simulink model "FSAC2021_V1_Running"  (R2014a)
settings: Solver=FixedStepDiscrete  StartTime=0.0  StopTime=inf  FixedStep=0.0005  RelTol=1e-3
model workspace (MAT data in the model file):
  MCOS : class17 (value not decoded)
  MCOS : class17 (value not decoded)
  MCOS : class17 (value not decoded)
  MCOS : class17 (value not decoded)
  MCOS : class17 (value not decoded)
  MCOS : class17 (value not decoded)
  MCOS : class17 (value not decoded)
  MCOS : class17 (value not decoded)
  MCOS : class17 (value not decoded)
  MCOS : class17 (value not decoded)
  MCOS : class17 (value not decoded)
  MCOS : class17 (value not decoded)
  MCOS : class17 (value not decoded)
  MCOS : class17 (value not decoded)
  MCOS : class17 (value not decoded)
  MCOS : class17 (value not decoded)
  MCOS : class17 (value not decoded)
  MCOS : class17 (value not decoded)
  MCOS : class17 (value not decoded)
  BUZZER_START = 1
  MCOS : class17 (value not decoded)
  MCOS : class17 (value not decoded)
  MCOS : class17 (value not decoded)
  MCOS : class17 (value not decoded)
  MCOS : class17 (value not decoded)
  MCOS : class17 (value not decoded)
  MCOS : class17 (value not decoded)
  MCOS : class17 (value not decoded)
  MCOS : class17 (value not decoded)
  MCOS : class17 (value not decoded)
  MCOS : class17 (value not decoded)
  MCOS : class17 (value not decoded)
  MCOS : class17 (value not decoded)
  MCOS : class17 (value not decoded)
  MCOS : class17 (value not decoded)
  MCOS : class17 (value not decoded)
  MCOS : class17 (value not decoded)
  MCOS : class17 (value not decoded)
  MCOS : class17 (value not decoded)
  MCOS : class17 (value not decoded)
  MCOS : class17 (value not decoded)
  MCOS : class17 (value not decoded)
  MCOS : class17 (value not decoded)
  MCOS : class17 (value not decoded)
  MCOS : class17 (value not decoded)
  MCOS : class17 (value not decoded)
  MCOS : class17 (value not decoded)
  MCOS : class17 (value not decoded)
  MCOS : class17 (value not decoded)
  MCOS : class17 (value not decoded)
  MCOS : class17 (value not decoded)
  MCOS : class17 (value not decoded)
  MCOS : class17 (value not decoded)
  MCOS : class17 (value not decoded)
  MCOS : class17 (value not decoded)
  MCOS : class17 (value not decoded)
  MCOS : class17 (value not decoded)
  MCOS : class17 (value not decoded)
  Brake = 11
  MCOS : class17 (value not decoded)
  MCOS : class17 (value not decoded)
  MCOS : class17 (value not decoded)
  MCOS : class17 (value not decoded)
  MCOS : class17 (value not decoded)
  MCOS : class17 (value not decoded)
  MCOS : class17 (value not decoded)
  MCOS : class17 (value not decoded)
  Sensor_Acc_b = 101.85
  Sensor_Acc_k = -0.0185
  Str_Sen_Orig_Angle = -341
  MCOS : class17 (value not decoded)
  Tire_D = 0.47
  T = 0.05
libraries: simulink x402, ec55xxlib x134
(part 15 of 17)

== system FSAC2021_V1_Running/ROUTING/TO_DCAN/Subsystem/DIAG_SCU/Operation_Enabled ==
  Operation_Enabled : Inport
  Operation_EnabledRon : Rounding  Operator=round
  Operation_Enabled_1sat : Saturate  UpperLimit=16  LowerLimit=0
  Operation_Enabled_Convert : DataTypeConversion  OutDataTypeStr=uint8
  Operation_Enabled_Convert1 : DataTypeConversion  OutDataTypeStr=uint32
  Operation_Enabled_D : Product  Inputs=*/
  Operation_Enabled_F : Constant  OutDataTypeStr=single
  Operation_Enabled_L : simulink/Logic and Bit Operations/Bitwise Operator  logicop=AND  UseBitMask=on  BitMask=16  BitMaskRealWorld=Stored Integer
  Operation_Enabled_O : Constant  Value=0  OutDataTypeStr=single
  Operation_Enabled_S : ArithShift  BitShiftNumber=-4
  Operation_Enabled_sat : Saturate  UpperLimit=0  LowerLimit=0
  Operation_Enabled_st : Sum  Inputs=+-
  output5 : Outport
  wires:
  Operation_Enabled/1 -> Operation_Enabled_sat/1
  Operation_Enabled_sat/1 -> Operation_Enabled_st/1
  Operation_Enabled_O/1 -> Operation_Enabled_st/2
  Operation_Enabled_st/1 -> Operation_Enabled_D/1
  Operation_Enabled_F/1 -> Operation_Enabled_D/2
  Operation_Enabled_D/1 -> Operation_EnabledRon/1
  Operation_EnabledRon/1 -> Operation_Enabled_S/1
  Operation_Enabled_S/1 -> Operation_Enabled_1sat/1
  Operation_Enabled_1sat/1 -> Operation_Enabled_Convert1/1
  Operation_Enabled_Convert1/1 -> Operation_Enabled_L/1
  Operation_Enabled_L/1 -> Operation_Enabled_Convert/1
  Operation_Enabled_Convert/1 -> output5/1

== system FSAC2021_V1_Running/ROUTING/TO_DCAN/Subsystem/DIAG_SCU/Str_Ang ==
  Str_Ang : Inport
  Str_AngBitCov : DataTypeConversion  OutDataTypeStr=uint8
  Str_AngCOV : DataTypeConversion  OutDataTypeStr=uint8
  Str_AngRon : Rounding  Operator=round
  Str_Ang_1sat : Saturate  UpperLimit=65535  LowerLimit=0
  Str_Ang_And : simulink/Logic and Bit Operations/Bitwise Operator  logicop=AND  UseBitMask=off  NumInputPorts=2  BitMask=bin2dec('11011001')  BitMaskRealWorld=Stored Integer
  Str_Ang_And_C : Constant  Value=255  OutDataTypeStr=uint32
  Str_Ang_Convert : DataTypeConversion  OutDataTypeStr=uint32
  Str_Ang_D : Product  Inputs=*/
  Str_Ang_D1 : Product  Inputs=*/
  Str_Ang_F : Constant  OutDataTypeStr=single
  Str_Ang_L : simulink/Logic and Bit Operations/Bitwise Operator  logicop=AND  UseBitMask=on  BitMask=65535  BitMaskRealWorld=Stored Integer
  Str_Ang_O : Constant  Value=0  OutDataTypeStr=single
  Str_Ang_S : ArithShift
  Str_Ang_sat : Saturate  UpperLimit=65535  LowerLimit=0
  Str_Ang_st : Sum  Inputs=+-
  Str_Angoutput2_C : Constant  Value=256
  output2 : Outport
  output3 : Outport  Port=2
  wires:
  Str_Ang/1 -> Str_Ang_sat/1
  Str_Ang_sat/1 -> Str_Ang_st/1
  Str_Ang_O/1 -> Str_Ang_st/2
  Str_Ang_st/1 -> Str_Ang_D/1
  Str_Ang_F/1 -> Str_Ang_D/2
  Str_Ang_D/1 -> Str_AngRon/1
  Str_AngRon/1 -> Str_Ang_S/1
  Str_Ang_S/1 -> Str_Ang_1sat/1
  Str_Ang_1sat/1 -> Str_Ang_Convert/1
  Str_Ang_Convert/1 -> Str_Ang_L/1
  Str_Ang_L/1 -> Str_Ang_D1/1, Str_Ang_And/1
  Str_Angoutput2_C/1 -> Str_Ang_D1/2
  Str_Ang_D1/1 -> Str_AngCOV/1
  Str_AngCOV/1 -> output2/1
  Str_Ang_And_C/1 -> Str_Ang_And/2
  Str_Ang_And/1 -> Str_AngBitCov/1
  Str_AngBitCov/1 -> output3/1

== system FSAC2021_V1_Running/ROUTING/TO_DCAN/Subsystem/DIAG_SCU/Str_Curr_Error_Fault ==
  Str_Curr_Error_Fault : Inport
  Str_Curr_Error_FaultRon : Rounding  Operator=round
  Str_Curr_Error_Fault_1sat : Saturate  UpperLimit=32  LowerLimit=0
  Str_Curr_Error_Fault_Convert : DataTypeConversion  OutDataTypeStr=uint8
  Str_Curr_Error_Fault_Convert1 : DataTypeConversion  OutDataTypeStr=uint32
  Str_Curr_Error_Fault_D : Product  Inputs=*/
  Str_Curr_Error_Fault_F : Constant  OutDataTypeStr=single
  Str_Curr_Error_Fault_L : simulink/Logic and Bit Operations/Bitwise Operator  logicop=AND  UseBitMask=on  BitMask=32  BitMaskRealWorld=Stored Integer
  Str_Curr_Error_Fault_O : Constant  Value=0  OutDataTypeStr=single
  Str_Curr_Error_Fault_S : ArithShift  BitShiftNumber=-5
  Str_Curr_Error_Fault_sat : Saturate  UpperLimit=0  LowerLimit=0
  Str_Curr_Error_Fault_st : Sum  Inputs=+-
  output7 : Outport
  wires:
  Str_Curr_Error_Fault/1 -> Str_Curr_Error_Fault_sat/1
  Str_Curr_Error_Fault_sat/1 -> Str_Curr_Error_Fault_st/1
  Str_Curr_Error_Fault_O/1 -> Str_Curr_Error_Fault_st/2
  Str_Curr_Error_Fault_st/1 -> Str_Curr_Error_Fault_D/1
  Str_Curr_Error_Fault_F/1 -> Str_Curr_Error_Fault_D/2
  Str_Curr_Error_Fault_D/1 -> Str_Curr_Error_FaultRon/1
  Str_Curr_Error_FaultRon/1 -> Str_Curr_Error_Fault_S/1
  Str_Curr_Error_Fault_S/1 -> Str_Curr_Error_Fault_1sat/1
  Str_Curr_Error_Fault_1sat/1 -> Str_Curr_Error_Fault_Convert1/1
  Str_Curr_Error_Fault_Convert1/1 -> Str_Curr_Error_Fault_L/1
  Str_Curr_Error_Fault_L/1 -> Str_Curr_Error_Fault_Convert/1
  Str_Curr_Error_Fault_Convert/1 -> output7/1

== system FSAC2021_V1_Running/ROUTING/TO_DCAN/Subsystem/DIAG_SCU/Str_Current ==
  Str_Current : Inport
  Str_CurrentABS : Abs
  Str_CurrentCS : ArithShift  BitShiftNumber=-8
  Str_CurrentConS : Constant  OutDataTypeStr=single
  Str_CurrentCosR : Constant  Value=0  OutDataTypeStr=uint8
  Str_CurrentROP : RelationalOperator  Operator=<  OutDataTypeStr=boolean
  Str_CurrentRon : Rounding  Operator=round
  Str_CurrentSW : Switch  Criteria=u2 ~= 0
  Str_Current_1sat : Saturate  UpperLimit=255  LowerLimit=0
  Str_Current_Convert : DataTypeConversion  OutDataTypeStr=uint8
  Str_Current_Convert1 : DataTypeConversion  OutDataTypeStr=uint32
  Str_Current_D : Product  Inputs=*/
  Str_Current_F : Constant  OutDataTypeStr=single
  Str_Current_L : simulink/Logic and Bit Operations/Bitwise Operator  logicop=AND  UseBitMask=on  BitMask=255  BitMaskRealWorld=Stored Integer
  Str_Current_O : Constant  Value=0  OutDataTypeStr=single
  Str_Current_S : ArithShift
  Str_Current_sat : Saturate  UpperLimit=127  LowerLimit=-128
  Str_Current_st : Sum  Inputs=+-
  Str_Currentsubcon : Sum  Inputs=+-
  output4 : Outport
  wires:
  Str_Current/1 -> Str_Current_sat/1
  Str_Current_sat/1 -> Str_Current_st/1
  Str_Current_O/1 -> Str_Current_st/2
  Str_Current_st/1 -> Str_Current_D/1
  Str_Current_F/1 -> Str_Current_D/2
  Str_Current_D/1 -> Str_CurrentRon/1
  Str_CurrentRon/1 -> Str_CurrentROP/1, Str_CurrentABS/1, Str_CurrentSW/3
  Str_CurrentCosR/1 -> Str_CurrentROP/2
  Str_CurrentConS/1 -> Str_CurrentCS/1
  Str_CurrentCS/1 -> Str_Currentsubcon/1
  Str_CurrentABS/1 -> Str_Currentsubcon/2
  Str_Currentsubcon/1 -> Str_CurrentSW/1
  Str_CurrentROP/1 -> Str_CurrentSW/2
  Str_CurrentSW/1 -> Str_Current_S/1
  Str_Current_S/1 -> Str_Current_1sat/1
  Str_Current_1sat/1 -> Str_Current_Convert1/1
  Str_Current_Convert1/1 -> Str_Current_L/1
  Str_Current_L/1 -> Str_Current_Convert/1
  Str_Current_Convert/1 -> output4/1

== system FSAC2021_V1_Running/ROUTING/TO_DCAN/Subsystem/DIAG_SCU/Str_Deg ==
  Str_Deg : Inport
  Str_DegABS : Abs
  Str_DegCS : ArithShift  BitShiftNumber=-8
  Str_DegConS : Constant  OutDataTypeStr=single
  Str_DegCosR : Constant  Value=0  OutDataTypeStr=uint8
  Str_DegROP : RelationalOperator  Operator=<  OutDataTypeStr=boolean
  Str_DegRon : Rounding  Operator=round
  Str_DegSW : Switch  Criteria=u2 ~= 0
  Str_Deg_1sat : Saturate  UpperLimit=255  LowerLimit=0
  Str_Deg_Convert : DataTypeConversion  OutDataTypeStr=uint8
  Str_Deg_Convert1 : DataTypeConversion  OutDataTypeStr=uint32
  Str_Deg_D : Product  Inputs=*/
  Str_Deg_F : Constant  OutDataTypeStr=single
  Str_Deg_L : simulink/Logic and Bit Operations/Bitwise Operator  logicop=AND  UseBitMask=on  BitMask=255  BitMaskRealWorld=Stored Integer
  Str_Deg_O : Constant  Value=0  OutDataTypeStr=single
  Str_Deg_S : ArithShift
  Str_Deg_sat : Saturate  UpperLimit=120  LowerLimit=-120
  Str_Deg_st : Sum  Inputs=+-
  Str_Degsubcon : Sum  Inputs=+-
  output1 : Outport
  wires:
  Str_Deg/1 -> Str_Deg_sat/1
  Str_Deg_sat/1 -> Str_Deg_st/1
  Str_Deg_O/1 -> Str_Deg_st/2
  Str_Deg_st/1 -> Str_Deg_D/1
  Str_Deg_F/1 -> Str_Deg_D/2
  Str_Deg_D/1 -> Str_DegRon/1
  Str_DegRon/1 -> Str_DegROP/1, Str_DegABS/1, Str_DegSW/3
  Str_DegCosR/1 -> Str_DegROP/2
  Str_DegConS/1 -> Str_DegCS/1
  Str_DegCS/1 -> Str_Degsubcon/1
  Str_DegABS/1 -> Str_Degsubcon/2
  Str_Degsubcon/1 -> Str_DegSW/1
  Str_DegROP/1 -> Str_DegSW/2
  Str_DegSW/1 -> Str_Deg_S/1
  Str_Deg_S/1 -> Str_Deg_1sat/1
  Str_Deg_1sat/1 -> Str_Deg_Convert1/1
  Str_Deg_Convert1/1 -> Str_Deg_L/1
  Str_Deg_L/1 -> Str_Deg_Convert/1
  Str_Deg_Convert/1 -> output1/1

== system FSAC2021_V1_Running/ROUTING/TO_DCAN/Subsystem/DIAG_SCU/Str_Encoder_Error ==
  Str_Encoder_Error : Inport
  Str_Encoder_ErrorRon : Rounding  Operator=round
  Str_Encoder_Error_1sat : Saturate  UpperLimit=16  LowerLimit=0
  Str_Encoder_Error_Convert : DataTypeConversion  OutDataTypeStr=uint8
  Str_Encoder_Error_Convert1 : DataTypeConversion  OutDataTypeStr=uint32
  Str_Encoder_Error_D : Product  Inputs=*/
  Str_Encoder_Error_F : Constant  OutDataTypeStr=single
  Str_Encoder_Error_L : simulink/Logic and Bit Operations/Bitwise Operator  logicop=AND  UseBitMask=on  BitMask=16  BitMaskRealWorld=Stored Integer
  Str_Encoder_Error_O : Constant  Value=0  OutDataTypeStr=single
  Str_Encoder_Error_S : ArithShift  BitShiftNumber=-4
  Str_Encoder_Error_sat : Saturate  UpperLimit=0  LowerLimit=0
  Str_Encoder_Error_st : Sum  Inputs=+-
  output6 : Outport
  wires:
  Str_Encoder_Error/1 -> Str_Encoder_Error_sat/1
  Str_Encoder_Error_sat/1 -> Str_Encoder_Error_st/1
  Str_Encoder_Error_O/1 -> Str_Encoder_Error_st/2
  Str_Encoder_Error_st/1 -> Str_Encoder_Error_D/1
  Str_Encoder_Error_F/1 -> Str_Encoder_Error_D/2
  Str_Encoder_Error_D/1 -> Str_Encoder_ErrorRon/1
  Str_Encoder_ErrorRon/1 -> Str_Encoder_Error_S/1
  Str_Encoder_Error_S/1 -> Str_Encoder_Error_1sat/1
  Str_Encoder_Error_1sat/1 -> Str_Encoder_Error_Convert1/1
  Str_Encoder_Error_Convert1/1 -> Str_Encoder_Error_L/1
  Str_Encoder_Error_L/1 -> Str_Encoder_Error_Convert/1
  Str_Encoder_Error_Convert/1 -> output6/1

== system FSAC2021_V1_Running/ROUTING/TO_DCAN/Subsystem/DIAG_SCU/Str_Flash_Error ==
  Str_Flash_Error : Inport
  Str_Flash_ErrorRon : Rounding  Operator=round
  Str_Flash_Error_1sat : Saturate  UpperLimit=8  LowerLimit=0
  Str_Flash_Error_Convert : DataTypeConversion  OutDataTypeStr=uint8
  Str_Flash_Error_Convert1 : DataTypeConversion  OutDataTypeStr=uint32
  Str_Flash_Error_D : Product  Inputs=*/
  Str_Flash_Error_F : Constant  OutDataTypeStr=single
  Str_Flash_Error_L : simulink/Logic and Bit Operations/Bitwise Operator  logicop=AND  UseBitMask=on  BitMask=8  BitMaskRealWorld=Stored Integer
  Str_Flash_Error_O : Constant  Value=0  OutDataTypeStr=single
  Str_Flash_Error_S : ArithShift  BitShiftNumber=-3
  Str_Flash_Error_sat : Saturate  UpperLimit=0  LowerLimit=0
  Str_Flash_Error_st : Sum  Inputs=+-
  output6 : Outport
  wires:
  Str_Flash_Error/1 -> Str_Flash_Error_sat/1
  Str_Flash_Error_sat/1 -> Str_Flash_Error_st/1
  Str_Flash_Error_O/1 -> Str_Flash_Error_st/2
  Str_Flash_Error_st/1 -> Str_Flash_Error_D/1
  Str_Flash_Error_F/1 -> Str_Flash_Error_D/2
  Str_Flash_Error_D/1 -> Str_Flash_ErrorRon/1
  Str_Flash_ErrorRon/1 -> Str_Flash_Error_S/1
  Str_Flash_Error_S/1 -> Str_Flash_Error_1sat/1
  Str_Flash_Error_1sat/1 -> Str_Flash_Error_Convert1/1
  Str_Flash_Error_Convert1/1 -> Str_Flash_Error_L/1
  Str_Flash_Error_L/1 -> Str_Flash_Error_Convert/1
  Str_Flash_Error_Convert/1 -> output6/1

== system FSAC2021_V1_Running/ROUTING/TO_DCAN/Subsystem/DIAG_SCU/Str_I2t_Alarm ==
  Str_I2t_Alarm : Inport
  Str_I2t_AlarmRon : Rounding  Operator=round
  Str_I2t_Alarm_1sat : Saturate  UpperLimit=1  LowerLimit=0
  Str_I2t_Alarm_Convert : DataTypeConversion  OutDataTypeStr=uint8
  Str_I2t_Alarm_Convert1 : DataTypeConversion  OutDataTypeStr=uint32
  Str_I2t_Alarm_D : Product  Inputs=*/
  Str_I2t_Alarm_F : Constant  OutDataTypeStr=single
  Str_I2t_Alarm_L : simulink/Logic and Bit Operations/Bitwise Operator  logicop=AND  UseBitMask=on  BitMask=1  BitMaskRealWorld=Stored Integer
  Str_I2t_Alarm_O : Constant  Value=0  OutDataTypeStr=single
  Str_I2t_Alarm_S : ArithShift
  Str_I2t_Alarm_sat : Saturate  UpperLimit=0  LowerLimit=0
  Str_I2t_Alarm_st : Sum  Inputs=+-
  output5 : Outport
  wires:
  Str_I2t_Alarm/1 -> Str_I2t_Alarm_sat/1
  Str_I2t_Alarm_sat/1 -> Str_I2t_Alarm_st/1
  Str_I2t_Alarm_O/1 -> Str_I2t_Alarm_st/2
  Str_I2t_Alarm_st/1 -> Str_I2t_Alarm_D/1
  Str_I2t_Alarm_F/1 -> Str_I2t_Alarm_D/2
  Str_I2t_Alarm_D/1 -> Str_I2t_AlarmRon/1
  Str_I2t_AlarmRon/1 -> Str_I2t_Alarm_S/1
  Str_I2t_Alarm_S/1 -> Str_I2t_Alarm_1sat/1
  Str_I2t_Alarm_1sat/1 -> Str_I2t_Alarm_Convert1/1
  Str_I2t_Alarm_Convert1/1 -> Str_I2t_Alarm_L/1
  Str_I2t_Alarm_L/1 -> Str_I2t_Alarm_Convert/1
  Str_I2t_Alarm_Convert/1 -> output5/1

== system FSAC2021_V1_Running/ROUTING/TO_DCAN/Subsystem/DIAG_SCU/Str_I2t_Warning ==
  Str_I2t_Warning : Inport
  Str_I2t_WarningRon : Rounding  Operator=round
  Str_I2t_Warning_1sat : Saturate  UpperLimit=2  LowerLimit=0
  Str_I2t_Warning_Convert : DataTypeConversion  OutDataTypeStr=uint8
  Str_I2t_Warning_Convert1 : DataTypeConversion  OutDataTypeStr=uint32
  Str_I2t_Warning_D : Product  Inputs=*/
  Str_I2t_Warning_F : Constant  OutDataTypeStr=single
  Str_I2t_Warning_L : simulink/Logic and Bit Operations/Bitwise Operator  logicop=AND  UseBitMask=on  BitMask=2  BitMaskRealWorld=Stored Integer
  Str_I2t_Warning_O : Constant  Value=0  OutDataTypeStr=single
  Str_I2t_Warning_S : ArithShift  BitShiftNumber=-1
  Str_I2t_Warning_sat : Saturate  UpperLimit=0  LowerLimit=0
  Str_I2t_Warning_st : Sum  Inputs=+-
  output5 : Outport
  wires:
  Str_I2t_Warning/1 -> Str_I2t_Warning_sat/1
  Str_I2t_Warning_sat/1 -> Str_I2t_Warning_st/1
  Str_I2t_Warning_O/1 -> Str_I2t_Warning_st/2
  Str_I2t_Warning_st/1 -> Str_I2t_Warning_D/1
  Str_I2t_Warning_F/1 -> Str_I2t_Warning_D/2
  Str_I2t_Warning_D/1 -> Str_I2t_WarningRon/1
  Str_I2t_WarningRon/1 -> Str_I2t_Warning_S/1
  Str_I2t_Warning_S/1 -> Str_I2t_Warning_1sat/1
  Str_I2t_Warning_1sat/1 -> Str_I2t_Warning_Convert1/1
  Str_I2t_Warning_Convert1/1 -> Str_I2t_Warning_L/1
  Str_I2t_Warning_L/1 -> Str_I2t_Warning_Convert/1
  Str_I2t_Warning_Convert/1 -> output5/1

== system FSAC2021_V1_Running/ROUTING/TO_DCAN/Subsystem/DIAG_SCU/Str_Limit_Pos_Alarm ==
  Str_Limit_Pos_Alarm : Inport
  Str_Limit_Pos_AlarmRon : Rounding  Operator=round
  Str_Limit_Pos_Alarm_1sat : Saturate  UpperLimit=2  LowerLimit=0
  Str_Limit_Pos_Alarm_Convert : DataTypeConversion  OutDataTypeStr=uint8
  Str_Limit_Pos_Alarm_Convert1 : DataTypeConversion  OutDataTypeStr=uint32
  Str_Limit_Pos_Alarm_D : Product  Inputs=*/
  Str_Limit_Pos_Alarm_F : Constant  OutDataTypeStr=single
  Str_Limit_Pos_Alarm_L : simulink/Logic and Bit Operations/Bitwise Operator  logicop=AND  UseBitMask=on  BitMask=2  BitMaskRealWorld=Stored Integer
  Str_Limit_Pos_Alarm_O : Constant  Value=0  OutDataTypeStr=single
  Str_Limit_Pos_Alarm_S : ArithShift  BitShiftNumber=-1
  Str_Limit_Pos_Alarm_sat : Saturate  UpperLimit=0  LowerLimit=0
  Str_Limit_Pos_Alarm_st : Sum  Inputs=+-
  output6 : Outport
  wires:
  Str_Limit_Pos_Alarm/1 -> Str_Limit_Pos_Alarm_sat/1
  Str_Limit_Pos_Alarm_sat/1 -> Str_Limit_Pos_Alarm_st/1
  Str_Limit_Pos_Alarm_O/1 -> Str_Limit_Pos_Alarm_st/2
  Str_Limit_Pos_Alarm_st/1 -> Str_Limit_Pos_Alarm_D/1
  Str_Limit_Pos_Alarm_F/1 -> Str_Limit_Pos_Alarm_D/2
  Str_Limit_Pos_Alarm_D/1 -> Str_Limit_Pos_AlarmRon/1
  Str_Limit_Pos_AlarmRon/1 -> Str_Limit_Pos_Alarm_S/1
  Str_Limit_Pos_Alarm_S/1 -> Str_Limit_Pos_Alarm_1sat/1
  Str_Limit_Pos_Alarm_1sat/1 -> Str_Limit_Pos_Alarm_Convert1/1
  Str_Limit_Pos_Alarm_Convert1/1 -> Str_Limit_Pos_Alarm_L/1
  Str_Limit_Pos_Alarm_L/1 -> Str_Limit_Pos_Alarm_Convert/1
  Str_Limit_Pos_Alarm_Convert/1 -> output6/1

== system FSAC2021_V1_Running/ROUTING/TO_DCAN/Subsystem/DIAG_SCU/Str_Over_PosError ==
  Str_Over_PosError : Inport
  Str_Over_PosErrorRon : Rounding  Operator=round
  Str_Over_PosError_1sat : Saturate  UpperLimit=64  LowerLimit=0
  Str_Over_PosError_Convert : DataTypeConversion  OutDataTypeStr=uint8
  Str_Over_PosError_Convert1 : DataTypeConversion  OutDataTypeStr=uint32
  Str_Over_PosError_D : Product  Inputs=*/
  Str_Over_PosError_F : Constant  OutDataTypeStr=single
  Str_Over_PosError_L : simulink/Logic and Bit Operations/Bitwise Operator  logicop=AND  UseBitMask=on  BitMask=64  BitMaskRealWorld=Stored Integer
  Str_Over_PosError_O : Constant  Value=0  OutDataTypeStr=single
  Str_Over_PosError_S : ArithShift  BitShiftNumber=-6
  Str_Over_PosError_sat : Saturate  UpperLimit=0  LowerLimit=0
  Str_Over_PosError_st : Sum  Inputs=+-
  output7 : Outport
  wires:
  Str_Over_PosError/1 -> Str_Over_PosError_sat/1
  Str_Over_PosError_sat/1 -> Str_Over_PosError_st/1
  Str_Over_PosError_O/1 -> Str_Over_PosError_st/2
  Str_Over_PosError_st/1 -> Str_Over_PosError_D/1
  Str_Over_PosError_F/1 -> Str_Over_PosError_D/2
  Str_Over_PosError_D/1 -> Str_Over_PosErrorRon/1
  Str_Over_PosErrorRon/1 -> Str_Over_PosError_S/1
  Str_Over_PosError_S/1 -> Str_Over_PosError_1sat/1
  Str_Over_PosError_1sat/1 -> Str_Over_PosError_Convert1/1
  Str_Over_PosError_Convert1/1 -> Str_Over_PosError_L/1
  Str_Over_PosError_L/1 -> Str_Over_PosError_Convert/1
  Str_Over_PosError_Convert/1 -> output7/1

== system FSAC2021_V1_Running/ROUTING/TO_DCAN/Subsystem/DIAG_SCU/Str_Over_SpdError ==
  Str_Over_SpdError : Inport
  Str_Over_SpdErrorRon : Rounding  Operator=round
  Str_Over_SpdError_1sat : Saturate  UpperLimit=1  LowerLimit=0
  Str_Over_SpdError_Convert : DataTypeConversion  OutDataTypeStr=uint8
  Str_Over_SpdError_Convert1 : DataTypeConversion  OutDataTypeStr=uint32
  Str_Over_SpdError_D : Product  Inputs=*/
  Str_Over_SpdError_F : Constant  OutDataTypeStr=single
  Str_Over_SpdError_L : simulink/Logic and Bit Operations/Bitwise Operator  logicop=AND  UseBitMask=on  BitMask=1  BitMaskRealWorld=Stored Integer
  Str_Over_SpdError_O : Constant  Value=0  OutDataTypeStr=single
  Str_Over_SpdError_S : ArithShift
  Str_Over_SpdError_sat : Saturate  UpperLimit=1  LowerLimit=0
  Str_Over_SpdError_st : Sum  Inputs=+-
  output6 : Outport
  wires:
  Str_Over_SpdError/1 -> Str_Over_SpdError_sat/1
  Str_Over_SpdError_sat/1 -> Str_Over_SpdError_st/1
  Str_Over_SpdError_O/1 -> Str_Over_SpdError_st/2
  Str_Over_SpdError_st/1 -> Str_Over_SpdError_D/1
  Str_Over_SpdError_F/1 -> Str_Over_SpdError_D/2
  Str_Over_SpdError_D/1 -> Str_Over_SpdErrorRon/1
  Str_Over_SpdErrorRon/1 -> Str_Over_SpdError_S/1
  Str_Over_SpdError_S/1 -> Str_Over_SpdError_1sat/1
  Str_Over_SpdError_1sat/1 -> Str_Over_SpdError_Convert1/1
  Str_Over_SpdError_Convert1/1 -> Str_Over_SpdError_L/1
  Str_Over_SpdError_L/1 -> Str_Over_SpdError_Convert/1
  Str_Over_SpdError_Convert/1 -> output6/1

== system FSAC2021_V1_Running/ROUTING/TO_DCAN/Subsystem/DIAG_SCU/Str_Over_TopCurr ==
  Str_Over_TopCurr : Inport
  Str_Over_TopCurrRon : Rounding  Operator=round
  Str_Over_TopCurr_1sat : Saturate  UpperLimit=4  LowerLimit=0
  Str_Over_TopCurr_Convert : DataTypeConversion  OutDataTypeStr=uint8
  Str_Over_TopCurr_Convert1 : DataTypeConversion  OutDataTypeStr=uint32
  Str_Over_TopCurr_D : Product  Inputs=*/
  Str_Over_TopCurr_F : Constant  OutDataTypeStr=single
  Str_Over_TopCurr_L : simulink/Logic and Bit Operations/Bitwise Operator  logicop=AND  UseBitMask=on  BitMask=4  BitMaskRealWorld=Stored Integer
  Str_Over_TopCurr_O : Constant  Value=0  OutDataTypeStr=single
  Str_Over_TopCurr_S : ArithShift  BitShiftNumber=-2
  Str_Over_TopCurr_sat : Saturate  UpperLimit=0  LowerLimit=0
  Str_Over_TopCurr_st : Sum  Inputs=+-
  output6 : Outport
  wires:
  Str_Over_TopCurr/1 -> Str_Over_TopCurr_sat/1
  Str_Over_TopCurr_sat/1 -> Str_Over_TopCurr_st/1
  Str_Over_TopCurr_O/1 -> Str_Over_TopCurr_st/2
  Str_Over_TopCurr_st/1 -> Str_Over_TopCurr_D/1
  Str_Over_TopCurr_F/1 -> Str_Over_TopCurr_D/2
  Str_Over_TopCurr_D/1 -> Str_Over_TopCurrRon/1
  Str_Over_TopCurrRon/1 -> Str_Over_TopCurr_S/1
  Str_Over_TopCurr_S/1 -> Str_Over_TopCurr_1sat/1
  Str_Over_TopCurr_1sat/1 -> Str_Over_TopCurr_Convert1/1
  Str_Over_TopCurr_Convert1/1 -> Str_Over_TopCurr_L/1
  Str_Over_TopCurr_L/1 -> Str_Over_TopCurr_Convert/1
  Str_Over_TopCurr_Convert/1 -> output6/1

== system FSAC2021_V1_Running/ROUTING/TO_DCAN/Subsystem/DIAG_SCU/Str_Overvolt_Warning ==
  Str_Overvolt_Warning : Inport
  Str_Overvolt_WarningRon : Rounding  Operator=round
  Str_Overvolt_Warning_1sat : Saturate  UpperLimit=64  LowerLimit=0
  Str_Overvolt_Warning_Convert : DataTypeConversion  OutDataTypeStr=uint8
  Str_Overvolt_Warning_Convert1 : DataTypeConversion  OutDataTypeStr=uint32
  Str_Overvolt_Warning_D : Product  Inputs=*/
  Str_Overvolt_Warning_F : Constant  OutDataTypeStr=single
  Str_Overvolt_Warning_L : simulink/Logic and Bit Operations/Bitwise Operator  logicop=AND  UseBitMask=on  BitMask=64  BitMaskRealWorld=Stored Integer
  Str_Overvolt_Warning_O : Constant  Value=0  OutDataTypeStr=single
  Str_Overvolt_Warning_S : ArithShift  BitShiftNumber=-6
  Str_Overvolt_Warning_sat : Saturate  UpperLimit=0  LowerLimit=0
  Str_Overvolt_Warning_st : Sum  Inputs=+-
  output6 : Outport
  wires:
  Str_Overvolt_Warning/1 -> Str_Overvolt_Warning_sat/1
  Str_Overvolt_Warning_sat/1 -> Str_Overvolt_Warning_st/1
  Str_Overvolt_Warning_O/1 -> Str_Overvolt_Warning_st/2
  Str_Overvolt_Warning_st/1 -> Str_Overvolt_Warning_D/1
  Str_Overvolt_Warning_F/1 -> Str_Overvolt_Warning_D/2
  Str_Overvolt_Warning_D/1 -> Str_Overvolt_WarningRon/1
  Str_Overvolt_WarningRon/1 -> Str_Overvolt_Warning_S/1
  Str_Overvolt_Warning_S/1 -> Str_Overvolt_Warning_1sat/1
  Str_Overvolt_Warning_1sat/1 -> Str_Overvolt_Warning_Convert1/1
  Str_Overvolt_Warning_Convert1/1 -> Str_Overvolt_Warning_L/1
  Str_Overvolt_Warning_L/1 -> Str_Overvolt_Warning_Convert/1
  Str_Overvolt_Warning_Convert/1 -> output6/1

== system FSAC2021_V1_Running/ROUTING/TO_DCAN/Subsystem/DIAG_SCU/Str_Para_Error ==
  Str_Para_Error : Inport
  Str_Para_ErrorRon : Rounding  Operator=round
  Str_Para_Error_1sat : Saturate  UpperLimit=32  LowerLimit=0
  Str_Para_Error_Convert : DataTypeConversion  OutDataTypeStr=uint8
  Str_Para_Error_Convert1 : DataTypeConversion  OutDataTypeStr=uint32
  Str_Para_Error_D : Product  Inputs=*/
  Str_Para_Error_F : Constant  OutDataTypeStr=single
  Str_Para_Error_L : simulink/Logic and Bit Operations/Bitwise Operator  logicop=AND  UseBitMask=on  BitMask=32  BitMaskRealWorld=Stored Integer
  Str_Para_Error_O : Constant  Value=0  OutDataTypeStr=single
  Str_Para_Error_S : ArithShift  BitShiftNumber=-5
  Str_Para_Error_sat : Saturate  UpperLimit=0  LowerLimit=0
  Str_Para_Error_st : Sum  Inputs=+-
  output6 : Outport
  wires:
  Str_Para_Error/1 -> Str_Para_Error_sat/1
  Str_Para_Error_sat/1 -> Str_Para_Error_st/1
  Str_Para_Error_O/1 -> Str_Para_Error_st/2
  Str_Para_Error_st/1 -> Str_Para_Error_D/1
  Str_Para_Error_F/1 -> Str_Para_Error_D/2
  Str_Para_Error_D/1 -> Str_Para_ErrorRon/1
  Str_Para_ErrorRon/1 -> Str_Para_Error_S/1
  Str_Para_Error_S/1 -> Str_Para_Error_1sat/1
  Str_Para_Error_1sat/1 -> Str_Para_Error_Convert1/1
  Str_Para_Error_Convert1/1 -> Str_Para_Error_L/1
  Str_Para_Error_L/1 -> Str_Para_Error_Convert/1
  Str_Para_Error_Convert/1 -> output6/1

== system FSAC2021_V1_Running/ROUTING/TO_DCAN/Subsystem/DIAG_SCU/Str_PwrMod_TempHigh_Alarm ==
  Str_PwrMod_TempHigh_Alarm : Inport
  Str_PwrMod_TempHigh_AlarmRon : Rounding  Operator=round
  Str_PwrMod_TempHigh_Alarm_1sat : Saturate  UpperLimit=16  LowerLimit=0
  Str_PwrMod_TempHigh_Alarm_Convert : DataTypeConversion  OutDataTypeStr=uint8
  Str_PwrMod_TempHigh_Alarm_Convert1 : DataTypeConversion  OutDataTypeStr=uint32
  Str_PwrMod_TempHigh_Alarm_D : Product  Inputs=*/
  Str_PwrMod_TempHigh_Alarm_F : Constant  OutDataTypeStr=single
  Str_PwrMod_TempHigh_Alarm_L : simulink/Logic and Bit Operations/Bitwise Operator  logicop=AND  UseBitMask=on  BitMask=16  BitMaskRealWorld=Stored Integer
  Str_PwrMod_TempHigh_Alarm_O : Constant  Value=0  OutDataTypeStr=single
  Str_PwrMod_TempHigh_Alarm_S : ArithShift  BitShiftNumber=-4
  Str_PwrMod_TempHigh_Alarm_sat : Saturate  UpperLimit=1  LowerLimit=0
  Str_PwrMod_TempHigh_Alarm_st : Sum  Inputs=+-
  output7 : Outport
  wires:
  Str_PwrMod_TempHigh_Alarm/1 -> Str_PwrMod_TempHigh_Alarm_sat/1
  Str_PwrMod_TempHigh_Alarm_sat/1 -> Str_PwrMod_TempHigh_Alarm_st/1
  Str_PwrMod_TempHigh_Alarm_O/1 -> Str_PwrMod_TempHigh_Alarm_st/2
  Str_PwrMod_TempHigh_Alarm_st/1 -> Str_PwrMod_TempHigh_Alarm_D/1
  Str_PwrMod_TempHigh_Alarm_F/1 -> Str_PwrMod_TempHigh_Alarm_D/2
  Str_PwrMod_TempHigh_Alarm_D/1 -> Str_PwrMod_TempHigh_AlarmRon/1
  Str_PwrMod_TempHigh_AlarmRon/1 -> Str_PwrMod_TempHigh_Alarm_S/1
  Str_PwrMod_TempHigh_Alarm_S/1 -> Str_PwrMod_TempHigh_Alarm_1sat/1
  Str_PwrMod_TempHigh_Alarm_1sat/1 -> Str_PwrMod_TempHigh_Alarm_Convert1/1
  Str_PwrMod_TempHigh_Alarm_Convert1/1 -> Str_PwrMod_TempHigh_Alarm_L/1
  Str_PwrMod_TempHigh_Alarm_L/1 -> Str_PwrMod_TempHigh_Alarm_Convert/1
  Str_PwrMod_TempHigh_Alarm_Convert/1 -> output7/1

== system FSAC2021_V1_Running/ROUTING/TO_DCAN/Subsystem/DIAG_SCU/Str_PwrMod_TempHigh_Warning ==
  Str_PwrMod_TempHigh_Warning : Inport
  Str_PwrMod_TempHigh_WarningRon : Rounding  Operator=round
  Str_PwrMod_TempHigh_Warning_1sat : Saturate  UpperLimit=8  LowerLimit=0
  Str_PwrMod_TempHigh_Warning_Convert : DataTypeConversion  OutDataTypeStr=uint8
  Str_PwrMod_TempHigh_Warning_Convert1 : DataTypeConversion  OutDataTypeStr=uint32
  Str_PwrMod_TempHigh_Warning_D : Product  Inputs=*/
  Str_PwrMod_TempHigh_Warning_F : Constant  OutDataTypeStr=single
  Str_PwrMod_TempHigh_Warning_L : simulink/Logic and Bit Operations/Bitwise Operator  logicop=AND  UseBitMask=on  BitMask=8  BitMaskRealWorld=Stored Integer
  Str_PwrMod_TempHigh_Warning_O : Constant  Value=0  OutDataTypeStr=single
  Str_PwrMod_TempHigh_Warning_S : ArithShift  BitShiftNumber=-3
  Str_PwrMod_TempHigh_Warning_sat : Saturate  UpperLimit=1  LowerLimit=0
  Str_PwrMod_TempHigh_Warning_st : Sum  Inputs=+-
  output7 : Outport
  wires:
  Str_PwrMod_TempHigh_Warning/1 -> Str_PwrMod_TempHigh_Warning_sat/1
  Str_PwrMod_TempHigh_Warning_sat/1 -> Str_PwrMod_TempHigh_Warning_st/1
  Str_PwrMod_TempHigh_Warning_O/1 -> Str_PwrMod_TempHigh_Warning_st/2
  Str_PwrMod_TempHigh_Warning_st/1 -> Str_PwrMod_TempHigh_Warning_D/1
  Str_PwrMod_TempHigh_Warning_F/1 -> Str_PwrMod_TempHigh_Warning_D/2
  Str_PwrMod_TempHigh_Warning_D/1 -> Str_PwrMod_TempHigh_WarningRon/1
  Str_PwrMod_TempHigh_WarningRon/1 -> Str_PwrMod_TempHigh_Warning_S/1
  Str_PwrMod_TempHigh_Warning_S/1 -> Str_PwrMod_TempHigh_Warning_1sat/1
  Str_PwrMod_TempHigh_Warning_1sat/1 -> Str_PwrMod_TempHigh_Warning_Convert1/1
  Str_PwrMod_TempHigh_Warning_Convert1/1 -> Str_PwrMod_TempHigh_Warning_L/1
  Str_PwrMod_TempHigh_Warning_L/1 -> Str_PwrMod_TempHigh_Warning_Convert/1
  Str_PwrMod_TempHigh_Warning_Convert/1 -> output7/1

== system FSAC2021_V1_Running/ROUTING/TO_DCAN/Subsystem/DIAG_SCU/Str_Spd_Over_Alam ==
  Str_Spd_Over_Alam : Inport
  Str_Spd_Over_AlamRon : Rounding  Operator=round
  Str_Spd_Over_Alam_1sat : Saturate  UpperLimit=128  LowerLimit=0
  Str_Spd_Over_Alam_Convert : DataTypeConversion  OutDataTypeStr=uint8
  Str_Spd_Over_Alam_Convert1 : DataTypeConversion  OutDataTypeStr=uint32
  Str_Spd_Over_Alam_D : Product  Inputs=*/
  Str_Spd_Over_Alam_F : Constant  OutDataTypeStr=single
  Str_Spd_Over_Alam_L : simulink/Logic and Bit Operations/Bitwise Operator  logicop=AND  UseBitMask=on  BitMask=128  BitMaskRealWorld=Stored Integer
  Str_Spd_Over_Alam_O : Constant  Value=0  OutDataTypeStr=single
  Str_Spd_Over_Alam_S : ArithShift  BitShiftNumber=-7
  Str_Spd_Over_Alam_sat : Saturate  UpperLimit=0  LowerLimit=0
  Str_Spd_Over_Alam_st : Sum  Inputs=+-
  output7 : Outport
  wires:
  Str_Spd_Over_Alam/1 -> Str_Spd_Over_Alam_sat/1
  Str_Spd_Over_Alam_sat/1 -> Str_Spd_Over_Alam_st/1
  Str_Spd_Over_Alam_O/1 -> Str_Spd_Over_Alam_st/2
  Str_Spd_Over_Alam_st/1 -> Str_Spd_Over_Alam_D/1
  Str_Spd_Over_Alam_F/1 -> Str_Spd_Over_Alam_D/2
  Str_Spd_Over_Alam_D/1 -> Str_Spd_Over_AlamRon/1
  Str_Spd_Over_AlamRon/1 -> Str_Spd_Over_Alam_S/1
  Str_Spd_Over_Alam_S/1 -> Str_Spd_Over_Alam_1sat/1
  Str_Spd_Over_Alam_1sat/1 -> Str_Spd_Over_Alam_Convert1/1
  Str_Spd_Over_Alam_Convert1/1 -> Str_Spd_Over_Alam_L/1
  Str_Spd_Over_Alam_L/1 -> Str_Spd_Over_Alam_Convert/1
  Str_Spd_Over_Alam_Convert/1 -> output7/1

== system FSAC2021_V1_Running/ROUTING/TO_DCAN/Subsystem/DIAG_SCU/Str_System_Error ==
  Str_System_Error : Inport
  Str_System_ErrorRon : Rounding  Operator=round
  Str_System_Error_1sat : Saturate  UpperLimit=4  LowerLimit=0
  Str_System_Error_Convert : DataTypeConversion  OutDataTypeStr=uint8
  Str_System_Error_Convert1 : DataTypeConversion  OutDataTypeStr=uint32
  Str_System_Error_D : Product  Inputs=*/
  Str_System_Error_F : Constant  OutDataTypeStr=single
  Str_System_Error_L : simulink/Logic and Bit Operations/Bitwise Operator  logicop=AND  UseBitMask=on  BitMask=4  BitMaskRealWorld=Stored Integer
  Str_System_Error_O : Constant  Value=0  OutDataTypeStr=single
  Str_System_Error_S : ArithShift  BitShiftNumber=-2
  Str_System_Error_sat : Saturate  UpperLimit=0  LowerLimit=0
  Str_System_Error_st : Sum  Inputs=+-
  output5 : Outport
  wires:
  Str_System_Error/1 -> Str_System_Error_sat/1
  Str_System_Error_sat/1 -> Str_System_Error_st/1
  Str_System_Error_O/1 -> Str_System_Error_st/2
  Str_System_Error_st/1 -> Str_System_Error_D/1
  Str_System_Error_F/1 -> Str_System_Error_D/2
  Str_System_Error_D/1 -> Str_System_ErrorRon/1
  Str_System_ErrorRon/1 -> Str_System_Error_S/1
  Str_System_Error_S/1 -> Str_System_Error_1sat/1
  Str_System_Error_1sat/1 -> Str_System_Error_Convert1/1
  Str_System_Error_Convert1/1 -> Str_System_Error_L/1
  Str_System_Error_L/1 -> Str_System_Error_Convert/1
  Str_System_Error_Convert/1 -> output5/1

== system FSAC2021_V1_Running/ROUTING/TO_DCAN/Subsystem/DIAG_SCU/Str_UnderVolt_Warning ==
  Str_UnderVolt_Warning : Inport
  Str_UnderVolt_WarningRon : Rounding  Operator=round
  Str_UnderVolt_Warning_1sat : Saturate  UpperLimit=128  LowerLimit=0
  Str_UnderVolt_Warning_Convert : DataTypeConversion  OutDataTypeStr=uint8
  Str_UnderVolt_Warning_Convert1 : DataTypeConversion  OutDataTypeStr=uint32
  Str_UnderVolt_Warning_D : Product  Inputs=*/
  Str_UnderVolt_Warning_F : Constant  OutDataTypeStr=single
  Str_UnderVolt_Warning_L : simulink/Logic and Bit Operations/Bitwise Operator  logicop=AND  UseBitMask=on  BitMask=128  BitMaskRealWorld=Stored Integer
  Str_UnderVolt_Warning_O : Constant  Value=0  OutDataTypeStr=single
  Str_UnderVolt_Warning_S : ArithShift  BitShiftNumber=-7
  Str_UnderVolt_Warning_sat : Saturate  UpperLimit=0  LowerLimit=0
  Str_UnderVolt_Warning_st : Sum  Inputs=+-
  output6 : Outport
  wires:
  Str_UnderVolt_Warning/1 -> Str_UnderVolt_Warning_sat/1
  Str_UnderVolt_Warning_sat/1 -> Str_UnderVolt_Warning_st/1
  Str_UnderVolt_Warning_O/1 -> Str_UnderVolt_Warning_st/2
  Str_UnderVolt_Warning_st/1 -> Str_UnderVolt_Warning_D/1
  Str_UnderVolt_Warning_F/1 -> Str_UnderVolt_Warning_D/2
  Str_UnderVolt_Warning_D/1 -> Str_UnderVolt_WarningRon/1
  Str_UnderVolt_WarningRon/1 -> Str_UnderVolt_Warning_S/1
  Str_UnderVolt_Warning_S/1 -> Str_UnderVolt_Warning_1sat/1
  Str_UnderVolt_Warning_1sat/1 -> Str_UnderVolt_Warning_Convert1/1
  Str_UnderVolt_Warning_Convert1/1 -> Str_UnderVolt_Warning_L/1
  Str_UnderVolt_Warning_L/1 -> Str_UnderVolt_Warning_Convert/1
  Str_UnderVolt_Warning_Convert/1 -> output6/1

== system FSAC2021_V1_Running/ROUTING/TO_DCAN/Subsystem/DIAG_SCU/Swtiched_On ==
  Swtiched_On : Inport
  Swtiched_OnRon : Rounding  Operator=round
  Swtiched_On_1sat : Saturate  UpperLimit=128  LowerLimit=0
  Swtiched_On_Convert : DataTypeConversion  OutDataTypeStr=uint8
  Swtiched_On_Convert1 : DataTypeConversion  OutDataTypeStr=uint32
  Swtiched_On_D : Product  Inputs=*/
  Swtiched_On_F : Constant  OutDataTypeStr=single
  Swtiched_On_L : simulink/Logic and Bit Operations/Bitwise Operator  logicop=AND  UseBitMask=on  BitMask=128  BitMaskRealWorld=Stored Integer
  Swtiched_On_O : Constant  Value=0  OutDataTypeStr=single
  Swtiched_On_S : ArithShift  BitShiftNumber=-7
  Swtiched_On_sat : Saturate  UpperLimit=0  LowerLimit=0
  Swtiched_On_st : Sum  Inputs=+-
  output5 : Outport
  wires:
  Swtiched_On/1 -> Swtiched_On_sat/1
  Swtiched_On_sat/1 -> Swtiched_On_st/1
  Swtiched_On_O/1 -> Swtiched_On_st/2
  Swtiched_On_st/1 -> Swtiched_On_D/1
  Swtiched_On_F/1 -> Swtiched_On_D/2
  Swtiched_On_D/1 -> Swtiched_OnRon/1
  Swtiched_OnRon/1 -> Swtiched_On_S/1
  Swtiched_On_S/1 -> Swtiched_On_1sat/1
  Swtiched_On_1sat/1 -> Swtiched_On_Convert1/1
  Swtiched_On_Convert1/1 -> Swtiched_On_L/1
  Swtiched_On_L/1 -> Swtiched_On_Convert/1
  Swtiched_On_Convert/1 -> output5/1

== system FSAC2021_V1_Running/ROUTING/TO_DCAN/Subsystem/DIAG_SCU/Voltage_Enabled ==
  Voltage_Enabled : Inport
  Voltage_EnabledRon : Rounding  Operator=round
  Voltage_Enabled_1sat : Saturate  UpperLimit=8  LowerLimit=0
  Voltage_Enabled_Convert : DataTypeConversion  OutDataTypeStr=uint8
  Voltage_Enabled_Convert1 : DataTypeConversion  OutDataTypeStr=uint32
  Voltage_Enabled_D : Product  Inputs=*/
  Voltage_Enabled_F : Constant  OutDataTypeStr=single
  Voltage_Enabled_L : simulink/Logic and Bit Operations/Bitwise Operator  logicop=AND  UseBitMask=on  BitMask=8  BitMaskRealWorld=Stored Integer
  Voltage_Enabled_O : Constant  Value=0  OutDataTypeStr=single
  Voltage_Enabled_S : ArithShift  BitShiftNumber=-3
  Voltage_Enabled_sat : Saturate  UpperLimit=0  LowerLimit=0
  Voltage_Enabled_st : Sum  Inputs=+-
  output5 : Outport
  wires:
  Voltage_Enabled/1 -> Voltage_Enabled_sat/1
  Voltage_Enabled_sat/1 -> Voltage_Enabled_st/1
  Voltage_Enabled_O/1 -> Voltage_Enabled_st/2
  Voltage_Enabled_st/1 -> Voltage_Enabled_D/1
  Voltage_Enabled_F/1 -> Voltage_Enabled_D/2
  Voltage_Enabled_D/1 -> Voltage_EnabledRon/1
  Voltage_EnabledRon/1 -> Voltage_Enabled_S/1
  Voltage_Enabled_S/1 -> Voltage_Enabled_1sat/1
  Voltage_Enabled_1sat/1 -> Voltage_Enabled_Convert1/1
  Voltage_Enabled_Convert1/1 -> Voltage_Enabled_L/1
  Voltage_Enabled_L/1 -> Voltage_Enabled_Convert/1
  Voltage_Enabled_Convert/1 -> output5/1

== system FSAC2021_V1_Running/ROUTING/TO_DCAN/Subsystem/DIAG_SCU/Warning ==
  Warning : Inport
  WarningRon : Rounding  Operator=round
  Warning_1sat : Saturate  UpperLimit=64  LowerLimit=0
  Warning_Convert : DataTypeConversion  OutDataTypeStr=uint8
  Warning_Convert1 : DataTypeConversion  OutDataTypeStr=uint32
  Warning_D : Product  Inputs=*/
  Warning_F : Constant  OutDataTypeStr=single
  Warning_L : simulink/Logic and Bit Operations/Bitwise Operator  logicop=AND  UseBitMask=on  BitMask=64  BitMaskRealWorld=Stored Integer
  Warning_O : Constant  Value=0  OutDataTypeStr=single
  Warning_S : ArithShift  BitShiftNumber=-6
  Warning_sat : Saturate  UpperLimit=0  LowerLimit=0
  Warning_st : Sum  Inputs=+-
  output5 : Outport
  wires:
  Warning/1 -> Warning_sat/1
  Warning_sat/1 -> Warning_st/1
  Warning_O/1 -> Warning_st/2
  Warning_st/1 -> Warning_D/1
  Warning_F/1 -> Warning_D/2
  Warning_D/1 -> WarningRon/1
  WarningRon/1 -> Warning_S/1
  Warning_S/1 -> Warning_1sat/1
  Warning_1sat/1 -> Warning_Convert1/1
  Warning_Convert1/1 -> Warning_L/1
  Warning_L/1 -> Warning_Convert/1
  Warning_Convert/1 -> output5/1

== system FSAC2021_V1_Running/ROUTING/TO_DCAN/Subsystem/DIAG_VEH_INFO/AMI_State ==
  AMI_State : Inport
  AMI_StateRon : Rounding  Operator=round
  AMI_State_1sat : Saturate  UpperLimit=56  LowerLimit=0
  AMI_State_Convert : DataTypeConversion  OutDataTypeStr=uint8
  AMI_State_Convert1 : DataTypeConversion  OutDataTypeStr=uint32
  AMI_State_D : Product  Inputs=*/
  AMI_State_F : Constant  OutDataTypeStr=single
  AMI_State_L : simulink/Logic and Bit Operations/Bitwise Operator  logicop=AND  UseBitMask=on  BitMask=56  BitMaskRealWorld=Stored Integer
  AMI_State_O : Constant  Value=0  OutDataTypeStr=single
  AMI_State_S : ArithShift  BitShiftNumber=-3
  AMI_State_sat : Saturate  UpperLimit=7  LowerLimit=0
  AMI_State_st : Sum  Inputs=+-
  Constant{2..8} (7 alike) : Constant  Value=0  OutDataTypeStr=uint8  SampleTime=-1
  output1 : Outport
  output2 : Outport  Port=2
  output3 : Outport  Port=3
  output4 : Outport  Port=4
  output5 : Outport  Port=5
  output6 : Outport  Port=6
  output7 : Outport  Port=7
  output8 : Outport  Port=8
  wires:
  AMI_State/1 -> AMI_State_sat/1
  AMI_State_sat/1 -> AMI_State_st/1
  AMI_State_O/1 -> AMI_State_st/2
  AMI_State_st/1 -> AMI_State_D/1
  AMI_State_F/1 -> AMI_State_D/2
  AMI_State_D/1 -> AMI_StateRon/1
  AMI_StateRon/1 -> AMI_State_S/1
  AMI_State_S/1 -> AMI_State_1sat/1
  AMI_State_1sat/1 -> AMI_State_Convert1/1
  AMI_State_Convert1/1 -> AMI_State_L/1
  AMI_State_L/1 -> AMI_State_Convert/1
  AMI_State_Convert/1 -> output1/1
  Constant2/1 -> output2/1
  Constant3/1 -> output3/1
  Constant4/1 -> output4/1
  Constant5/1 -> output5/1
  Constant6/1 -> output6/1
  Constant7/1 -> output7/1
  Constant8/1 -> output8/1

== system FSAC2021_V1_Running/ROUTING/TO_DCAN/Subsystem/DIAG_VEH_INFO/ASMS_Swtich ==
  ASMS_Swtich : Inport
  ASMS_SwtichRon : Rounding  Operator=round
  ASMS_Swtich_1sat : Saturate  UpperLimit=4  LowerLimit=0
  ASMS_Swtich_Convert : DataTypeConversion  OutDataTypeStr=uint8
  ASMS_Swtich_Convert1 : DataTypeConversion  OutDataTypeStr=uint32
  ASMS_Swtich_D : Product  Inputs=*/
  ASMS_Swtich_F : Constant  OutDataTypeStr=single
  ASMS_Swtich_L : simulink/Logic and Bit Operations/Bitwise Operator  logicop=AND  UseBitMask=on  BitMask=4  BitMaskRealWorld=Stored Integer
  ASMS_Swtich_O : Constant  Value=0  OutDataTypeStr=single
  ASMS_Swtich_S : ArithShift  BitShiftNumber=-2
  ASMS_Swtich_sat : Saturate  UpperLimit=1  LowerLimit=0
  ASMS_Swtich_st : Sum  Inputs=+-
  Constant{1,3..8} (7 alike) : Constant  Value=0  OutDataTypeStr=uint8  SampleTime=-1
  output1 : Outport
  output2 : Outport  Port=2
  output3 : Outport  Port=3
  output4 : Outport  Port=4
  output5 : Outport  Port=5
  output6 : Outport  Port=6
  output7 : Outport  Port=7
  output8 : Outport  Port=8
  wires:
  ASMS_Swtich/1 -> ASMS_Swtich_sat/1
  ASMS_Swtich_sat/1 -> ASMS_Swtich_st/1
  ASMS_Swtich_O/1 -> ASMS_Swtich_st/2
  ASMS_Swtich_st/1 -> ASMS_Swtich_D/1
  ASMS_Swtich_F/1 -> ASMS_Swtich_D/2
  ASMS_Swtich_D/1 -> ASMS_SwtichRon/1
  ASMS_SwtichRon/1 -> ASMS_Swtich_S/1
  ASMS_Swtich_S/1 -> ASMS_Swtich_1sat/1
  ASMS_Swtich_1sat/1 -> ASMS_Swtich_Convert1/1
  ASMS_Swtich_Convert1/1 -> ASMS_Swtich_L/1
  ASMS_Swtich_L/1 -> ASMS_Swtich_Convert/1
  ASMS_Swtich_Convert/1 -> output2/1
  Constant1/1 -> output1/1
  Constant3/1 -> output3/1
  Constant4/1 -> output4/1
  Constant5/1 -> output5/1
  Constant6/1 -> output6/1
  Constant7/1 -> output7/1
  Constant8/1 -> output8/1

== system FSAC2021_V1_Running/ROUTING/TO_DCAN/Subsystem/DIAG_VEH_INFO/AS_State ==
  AS_State : Inport
  AS_StateRon : Rounding  Operator=round
  AS_State_1sat : Saturate  UpperLimit=7  LowerLimit=0
  AS_State_Convert : DataTypeConversion  OutDataTypeStr=uint8
  AS_State_Convert1 : DataTypeConversion  OutDataTypeStr=uint32
  AS_State_D : Product  Inputs=*/
  AS_State_F : Constant  OutDataTypeStr=single
  AS_State_L : simulink/Logic and Bit Operations/Bitwise Operator  logicop=AND  UseBitMask=on  BitMask=7  BitMaskRealWorld=Stored Integer
  AS_State_O : Constant  Value=0  OutDataTypeStr=single
  AS_State_S : ArithShift
  AS_State_sat : Saturate  UpperLimit=6  LowerLimit=0
  AS_State_st : Sum  Inputs=+-
  Constant{2..8} (7 alike) : Constant  Value=0  OutDataTypeStr=uint8  SampleTime=-1
  output1 : Outport
  output2 : Outport  Port=2
  output3 : Outport  Port=3
  output4 : Outport  Port=4
  output5 : Outport  Port=5
  output6 : Outport  Port=6
  output7 : Outport  Port=7
  output8 : Outport  Port=8
  wires:
  AS_State/1 -> AS_State_sat/1
  AS_State_sat/1 -> AS_State_st/1
  AS_State_O/1 -> AS_State_st/2
  AS_State_st/1 -> AS_State_D/1
  AS_State_F/1 -> AS_State_D/2
  AS_State_D/1 -> AS_StateRon/1
  AS_StateRon/1 -> AS_State_S/1
  AS_State_S/1 -> AS_State_1sat/1
  AS_State_1sat/1 -> AS_State_Convert1/1
  AS_State_Convert1/1 -> AS_State_L/1
  AS_State_L/1 -> AS_State_Convert/1
  AS_State_Convert/1 -> output1/1
  Constant2/1 -> output2/1
  Constant3/1 -> output3/1
  Constant4/1 -> output4/1
  Constant5/1 -> output5/1
  Constant6/1 -> output6/1
  Constant7/1 -> output7/1
  Constant8/1 -> output8/1

== system FSAC2021_V1_Running/ROUTING/TO_DCAN/Subsystem/DIAG_VEH_INFO/Acc_SN_1_Sts ==
  Acc_SN_1_Sts : Inport
  Acc_SN_1_StsRon : Rounding  Operator=round
  Acc_SN_1_Sts_1sat : Saturate  UpperLimit=128  LowerLimit=0
  Acc_SN_1_Sts_Convert : DataTypeConversion  OutDataTypeStr=uint8
  Acc_SN_1_Sts_Convert1 : DataTypeConversion  OutDataTypeStr=uint32
  Acc_SN_1_Sts_D : Product  Inputs=*/
  Acc_SN_1_Sts_F : Constant  OutDataTypeStr=single
  Acc_SN_1_Sts_L : simulink/Logic and Bit Operations/Bitwise Operator  logicop=AND  UseBitMask=on  BitMask=128  BitMaskRealWorld=Stored Integer
  Acc_SN_1_Sts_O : Constant  Value=0  OutDataTypeStr=single
  Acc_SN_1_Sts_S : ArithShift  BitShiftNumber=-7
  Acc_SN_1_Sts_sat : Saturate  UpperLimit=1  LowerLimit=0
  Acc_SN_1_Sts_st : Sum  Inputs=+-
  Constant{1..3,5..8} (7 alike) : Constant  Value=0  OutDataTypeStr=uint8  SampleTime=-1
  output1 : Outport
  output2 : Outport  Port=2
  output3 : Outport  Port=3
  output4 : Outport  Port=4
  output5 : Outport  Port=5
  output6 : Outport  Port=6
  output7 : Outport  Port=7
  output8 : Outport  Port=8
  wires:
  Acc_SN_1_Sts/1 -> Acc_SN_1_Sts_sat/1
  Acc_SN_1_Sts_sat/1 -> Acc_SN_1_Sts_st/1
  Acc_SN_1_Sts_O/1 -> Acc_SN_1_Sts_st/2
  Acc_SN_1_Sts_st/1 -> Acc_SN_1_Sts_D/1
  Acc_SN_1_Sts_F/1 -> Acc_SN_1_Sts_D/2
  Acc_SN_1_Sts_D/1 -> Acc_SN_1_StsRon/1
  Acc_SN_1_StsRon/1 -> Acc_SN_1_Sts_S/1
  Acc_SN_1_Sts_S/1 -> Acc_SN_1_Sts_1sat/1
  Acc_SN_1_Sts_1sat/1 -> Acc_SN_1_Sts_Convert1/1
  Acc_SN_1_Sts_Convert1/1 -> Acc_SN_1_Sts_L/1
  Acc_SN_1_Sts_L/1 -> Acc_SN_1_Sts_Convert/1
  Acc_SN_1_Sts_Convert/1 -> output4/1
  Constant1/1 -> output1/1
  Constant2/1 -> output2/1
  Constant3/1 -> output3/1
  Constant5/1 -> output5/1
  Constant6/1 -> output6/1
  Constant7/1 -> output7/1
  Constant8/1 -> output8/1

== system FSAC2021_V1_Running/ROUTING/TO_DCAN/Subsystem/DIAG_VEH_INFO/Acc_SN_2_Sts ==
  Acc_SN_2_Sts : Inport
  Acc_SN_2_StsRon : Rounding  Operator=round
  Acc_SN_2_Sts_1sat : Saturate  UpperLimit=64  LowerLimit=0
  Acc_SN_2_Sts_Convert : DataTypeConversion  OutDataTypeStr=uint8
  Acc_SN_2_Sts_Convert1 : DataTypeConversion  OutDataTypeStr=uint32
  Acc_SN_2_Sts_D : Product  Inputs=*/
  Acc_SN_2_Sts_F : Constant  OutDataTypeStr=single
  Acc_SN_2_Sts_L : simulink/Logic and Bit Operations/Bitwise Operator  logicop=AND  UseBitMask=on  BitMask=64  BitMaskRealWorld=Stored Integer
  Acc_SN_2_Sts_O : Constant  Value=0  OutDataTypeStr=single
  Acc_SN_2_Sts_S : ArithShift  BitShiftNumber=-6
  Acc_SN_2_Sts_sat : Saturate  UpperLimit=1  LowerLimit=0
  Acc_SN_2_Sts_st : Sum  Inputs=+-
  Constant{1..3,5..8} (7 alike) : Constant  Value=0  OutDataTypeStr=uint8  SampleTime=-1
  output1 : Outport
  output2 : Outport  Port=2
  output3 : Outport  Port=3
  output4 : Outport  Port=4
  output5 : Outport  Port=5
  output6 : Outport  Port=6
  output7 : Outport  Port=7
  output8 : Outport  Port=8
  wires:
  Acc_SN_2_Sts/1 -> Acc_SN_2_Sts_sat/1
  Acc_SN_2_Sts_sat/1 -> Acc_SN_2_Sts_st/1
  Acc_SN_2_Sts_O/1 -> Acc_SN_2_Sts_st/2
  Acc_SN_2_Sts_st/1 -> Acc_SN_2_Sts_D/1
  Acc_SN_2_Sts_F/1 -> Acc_SN_2_Sts_D/2
  Acc_SN_2_Sts_D/1 -> Acc_SN_2_StsRon/1
  Acc_SN_2_StsRon/1 -> Acc_SN_2_Sts_S/1
  Acc_SN_2_Sts_S/1 -> Acc_SN_2_Sts_1sat/1
  Acc_SN_2_Sts_1sat/1 -> Acc_SN_2_Sts_Convert1/1
  Acc_SN_2_Sts_Convert1/1 -> Acc_SN_2_Sts_L/1
  Acc_SN_2_Sts_L/1 -> Acc_SN_2_Sts_Convert/1
  Acc_SN_2_Sts_Convert/1 -> output4/1
  Constant1/1 -> output1/1
  Constant2/1 -> output2/1
  Constant3/1 -> output3/1
  Constant5/1 -> output5/1
  Constant6/1 -> output6/1
  Constant7/1 -> output7/1
  Constant8/1 -> output8/1

== system FSAC2021_V1_Running/ROUTING/TO_DCAN/Subsystem/DIAG_VEH_INFO/Brk_Disp_SN_Sts ==
  Brk_Disp_SN_Sts : Inport
  Brk_Disp_SN_StsRon : Rounding  Operator=round
  Brk_Disp_SN_Sts_1sat : Saturate  UpperLimit=32  LowerLimit=0
  Brk_Disp_SN_Sts_Convert : DataTypeConversion  OutDataTypeStr=uint8
  Brk_Disp_SN_Sts_Convert1 : DataTypeConversion  OutDataTypeStr=uint32
  Brk_Disp_SN_Sts_D : Product  Inputs=*/
  Brk_Disp_SN_Sts_F : Constant  OutDataTypeStr=single
  Brk_Disp_SN_Sts_L : simulink/Logic and Bit Operations/Bitwise Operator  logicop=AND  UseBitMask=on  BitMask=32  BitMaskRealWorld=Stored Integer
  Brk_Disp_SN_Sts_O : Constant  Value=0  OutDataTypeStr=single
  Brk_Disp_SN_Sts_S : ArithShift  BitShiftNumber=-5
  Brk_Disp_SN_Sts_sat : Saturate  UpperLimit=1  LowerLimit=0
  Brk_Disp_SN_Sts_st : Sum  Inputs=+-
  Constant{1..3,5..8} (7 alike) : Constant  Value=0  OutDataTypeStr=uint8  SampleTime=-1
  output1 : Outport
  output2 : Outport  Port=2
  output3 : Outport  Port=3
  output4 : Outport  Port=4
  output5 : Outport  Port=5
  output6 : Outport  Port=6
  output7 : Outport  Port=7
  output8 : Outport  Port=8
  wires:
  Brk_Disp_SN_Sts/1 -> Brk_Disp_SN_Sts_sat/1
  Brk_Disp_SN_Sts_sat/1 -> Brk_Disp_SN_Sts_st/1
  Brk_Disp_SN_Sts_O/1 -> Brk_Disp_SN_Sts_st/2
  Brk_Disp_SN_Sts_st/1 -> Brk_Disp_SN_Sts_D/1
  Brk_Disp_SN_Sts_F/1 -> Brk_Disp_SN_Sts_D/2
  Brk_Disp_SN_Sts_D/1 -> Brk_Disp_SN_StsRon/1
  Brk_Disp_SN_StsRon/1 -> Brk_Disp_SN_Sts_S/1
  Brk_Disp_SN_Sts_S/1 -> Brk_Disp_SN_Sts_1sat/1
  Brk_Disp_SN_Sts_1sat/1 -> Brk_Disp_SN_Sts_Convert1/1
  Brk_Disp_SN_Sts_Convert1/1 -> Brk_Disp_SN_Sts_L/1
  Brk_Disp_SN_Sts_L/1 -> Brk_Disp_SN_Sts_Convert/1
  Brk_Disp_SN_Sts_Convert/1 -> output4/1
  Constant1/1 -> output1/1
  Constant2/1 -> output2/1
  Constant3/1 -> output3/1
  Constant5/1 -> output5/1
  Constant6/1 -> output6/1
  Constant7/1 -> output7/1
  Constant8/1 -> output8/1
